simulink model "Motor"  (R2024a)
settings: Solver=VariableStepAuto  StartTime=0.0  StopTime=0.5  RelTol=1e-3
libraries: spsDetailedThyristorLib x4, spsMeanLib x3, spsCurrentMeasurementLib x2, spsVoltageMeasurementLib x2, spsACVoltageSourceLib x1, spsDCMachineLib x1, spsDCVoltageSourceLib x1, sps_lib x1
settings Model: Creator=yashg  LastModifiedBy=yashg
settings DataIOCC: ReturnWorkspaceOutputs=off

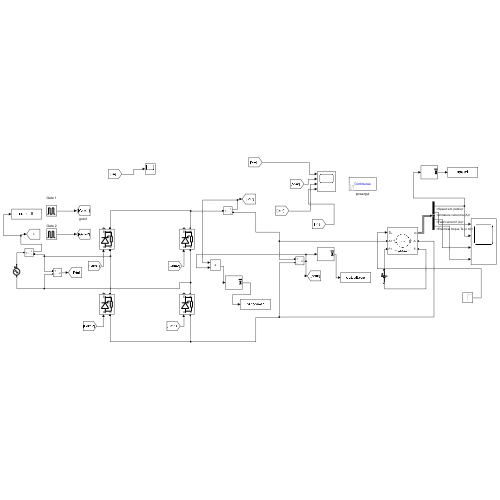
[thumbnail: Simulink's stored preview of the top-level diagram]
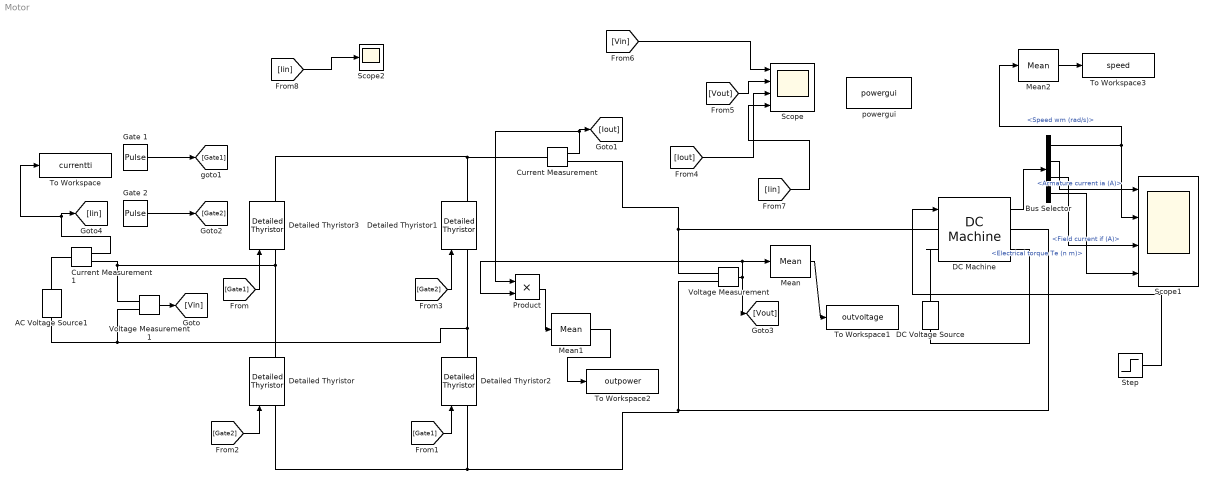
== system Motor ==
  AC Voltage Source1 : spsACVoltageSourceLib/AC Voltage Source  Amplitude=280  Phase=0  Frequency=50  SampleTime=0  Measurements=None  BusType=swing  Pref=10e3  Qref=0  Qmin=-inf  Qmax=+inf
  Bus Selector : BusSelector  OutputSignals=Speed wm (rad/s),Armature current ia (A),Field current if (A),Electrical torque Te (n m)
  Current Measurement : spsCurrentMeasurementLib/Current Measurement  PhasorSimulation=off  OutputType=Complex  PSBequivalent=0
  Current Measurement1 : spsCurrentMeasurementLib/Current Measurement  PhasorSimulation=off  OutputType=Complex  PSBequivalent=0
  DC Machine : spsDCMachineLib/DC Machine  PresetModel=02: 5HP 240V 1750RPM Field:150V  MechanicalLoad=Torque TL  FieldType=Wound  ShowDetailedParameters=on  MeasurementBus=off  RLa=[0.78 0.016]  RLf=[150 112.5]  Laf=1.234  MachineConstant=Torque constant (N.m/A)  Ke=1.8  Kt=1.8  J=0.05  Bm=0.01  Tf=0  w0=1  Ifinit=0.666666665186226  TsPowergui=0  TsBlock=-1
  DC Voltage Source : spsDCVoltageSourceLib/DC Voltage Source  Amplitude=100  Measurements=None
  Detailed Thyristor{,1..3} (4 alike) : spsDetailedThyristorLib/Detailed Thyristor  Ron=0.001  Lon=1e-3  Vf=0.8  IL=0.1  Tq=100e-6  IC=0  Rs=500  Cs=250e-9  Measurements=on
      settings: LibrarySourceBlock=sps_lib/Power Electronics/Detailed Thyristor
  "Gate 1 " : DiscretePulseGenerator  PulseType=Time based  Period=0.02  PulseWidth=50
  Gate 2 : DiscretePulseGenerator  PulseType=Time based  Period=0.02  PulseWidth=50  PhaseDelay=0.01
  Mean : spsMeanLib/Mean  Freq=60  Vinit=0  Ts=0
  Mean1 : spsMeanLib/Mean  Freq=60  Vinit=0  Ts=0
  Mean2 : spsMeanLib/Mean  Freq=60  Vinit=0  Ts=0
  Product : Product
  Scope : Scope  NumInputPorts=4
  Scope1 : Scope  NumInputPorts=4
  Scope2 : Scope
  Step : Step  Time=0  After=21.45  SampleTime=0
  To Workspace : ToWorkspace  VariableName=currentti  SaveFormat=Timeseries  SampleTime=-1
  To Workspace1 : ToWorkspace  VariableName=outvoltage  SampleTime=-1
      settings: MaxDataPoints=1
  To Workspace2 : ToWorkspace  VariableName=outpower  SampleTime=-1
      settings: MaxDataPoints=1
  To Workspace3 : ToWorkspace  VariableName=speed  SampleTime=-1
      settings: MaxDataPoints=1
  Voltage Measurement : spsVoltageMeasurementLib/Voltage Measurement  PhasorSimulation=off  OutputType=Complex  PSBequivalent=0
  Voltage Measurement1 : spsVoltageMeasurementLib/Voltage Measurement  PhasorSimulation=off  OutputType=Complex  PSBequivalent=0
  powergui : sps_lib/powergui  Priority=1  SimulationMode=Continuous  SampleTime=50e-6  frequency=60  Iterations=50  frequencyindice=50  Pbase=100e6  ErrMax=1e-4  UnitsV=kV  UnitsW=MW  buscounter=0  FunctionMessages=off  echomessages=off  EnableUseOfTLC=off  CurrentSourceSwitches=off  DisableSnubberDevices=off  DisableRonSwitches=off  DisableVfSwitches=off  DisplayEquations=off  AutomaticDiscreteSolvers=off  SolverType=Tustin/Backward Euler (TBE)  Interpol=off  ExternalGateDelay=off  methode=off  Ts=100  x0status=blocks  SPID=on  SwTol=0  HookPort=off  NonlinearTolerance=1e-4  nMaxIteration=100  ContinueOnMaxIteration=off  RestoreLinks=warning  ResistiveCurrentMeasurement=off  Frange=[0:2:500]  Ylog=off  Xlog=on  ShowGrid=off  save=off  variable=ZData  structure=0  ZoomFFT=off  StartTime=0.0  cycles=1  DisplayStyle=1  fundamental=60  FreqAxis=off  MaxFrequency=1000  frequencyindicesteady=1  RmsSteady=1  display=off
  wires:
  [Gate1] -> Detailed Thyristor2/1
  [Vout] -> Scope/2
  [Iout] -> Scope/3
  "Gate 1 "/1 -> [Gate1]
  Voltage Measurement/1 -> [Vout], Product/2, Mean/1
  Voltage Measurement1/1 -> [Vin]
  [Gate2] -> Detailed Thyristor1/1
  Gate 2/1 -> [Gate2]
  [Gate1] -> Detailed Thyristor3/1
  [Gate2] -> Detailed Thyristor/1
  [Vin] -> Scope/1
  Current Measurement/1 -> Product/1, [Iout]
  Current Measurement1/1 -> To Workspace/1, [Iin]
  [Iin] -> Scope/4
  Bus Selector/1 -> Scope1/2, Mean2/1  "<Speed wm (rad/s)>"
  DC Machine/1 -> Bus Selector/1
  Step/1 -> DC Machine/1
  [Iin] -> Scope2/1
  Mean/1 -> To Workspace1/1
  Product/1 -> Mean1/1
  Mean1/1 -> To Workspace2/1
  Mean2/1 -> To Workspace3/1
  Bus Selector/4 -> Scope1/4  "<Electrical torque Te (n m)>"
  Bus Selector/3 -> Scope1/3  "<Field current if (A)>"
  Bus Selector/2 -> Scope1/1  "<Armature current ia (A)>"
  connections:
  Voltage Measurement/LConn1 -- Current Measurement/RConn1 -- DC Machine/LConn1
  Detailed Thyristor3/LConn1 -- Voltage Measurement1/LConn1 -- Current Measurement1/RConn1 -- Detailed Thyristor/RConn1
  Detailed Thyristor2/RConn1 -- Detailed Thyristor1/LConn1 -- Voltage Measurement1/LConn2 -- AC Voltage Source1/LConn1
  Detailed Thyristor2/LConn1 -- DC Machine/RConn1 -- Voltage Measurement/LConn2 -- Detailed Thyristor/LConn1
  Detailed Thyristor3/RConn1 -- Detailed Thyristor1/RConn1 -- Current Measurement/LConn1
  Current Measurement1/LConn1 -- AC Voltage Source1/RConn1
  DC Machine/LConn2 -- DC Voltage Source/RConn1
  DC Machine/RConn2 -- DC Voltage Source/LConn1
